simulink model "test_dynamics_sim"  (R2021b)
settings: Solver=ode8  StartTime=0.0  StopTime=5000  FixedStep=0.01  RelTol=1e-3
values from neighbouring files (symbols this model uses):
  invJ = inv(J)    [test_dynamics1.m]    (also in test_dynamics2.m)
  Ir = 0    [test_dynamics1.m]    (also in test_dynamics2.m = 0.005)
  Ix = 0.0504    [test_dynamics1.m]    (also in test_dynamics2.m = 0.01)
  Iy = 0.0504    [test_dynamics1.m]    (also in test_dynamics2.m = 0.05)
  Iz = 0.0109    [test_dynamics1.m]    (also in test_dynamics2.m = 0.07)
  J = [Ix 0 0; 0 Iy 0; 0 0 Iz]    [test_dynamics1.m]    (also in test_dynamics2.m)
  Mx = 0    [test_dynamics2.m]
  My = 0    [test_dynamics2.m]
  Mz = 0    [test_dynamics2.m]
  omega0 = [omegax0, omegay0, omegaz0]'    [test_dynamics1.m]    (also in test_dynamics2.m)
  omegar = 0    [test_dynamics1.m]    (also in test_dynamics2.m = 6.28318530718)
  omegax0 = 0.45    [test_dynamics1.m]    (also in test_dynamics2.m = 1e-06)
  omegay0 = 0.52    [test_dynamics1.m]    (also in test_dynamics2.m = 1e-06)
  omegaz0 = 0.55    [test_dynamics1.m]    (also in test_dynamics2.m = 0.02)
  T_w = [0 0 0.0004]'    [test_dynamics2.m]
libraries: my_math_ops x3, vrlib x1
settings Model: Creator=Davide  LastModifiedBy=Davide
settings SolverCC: AlgebraicLoopSolver=TrustRegion
settings DebuggingCC: SFMachineParentedDataDiag=warning

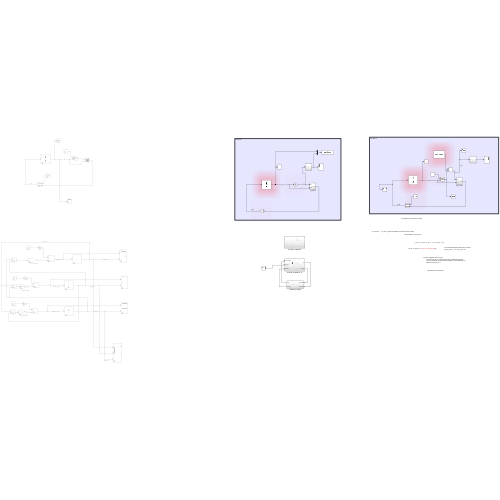
[thumbnail: Simulink's stored preview of the top-level diagram]
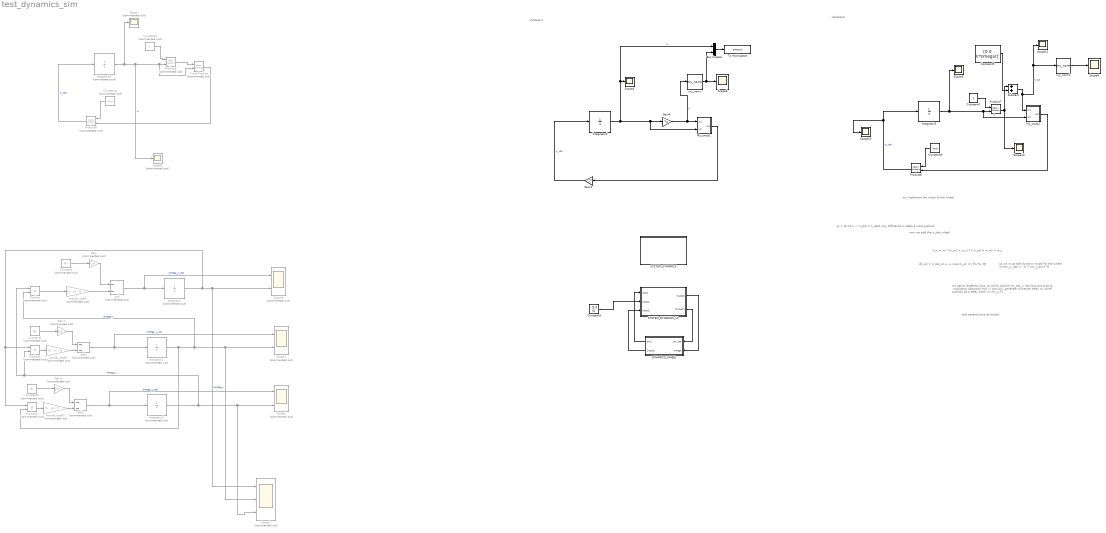
== system test_dynamics_sim ==
  note: Validator2
  note: Validator1
  note: add square wave as torque
  note: we get an algebraic loop, to solve:
      | explicit om_dot_z, rewriting but loosing ,modularity approach
      | trick in simulink, generate numerical delay on some quantity as a
      | delay block on om_z Z-1
  note: so we must add dynamic model for the wheel
      | Iw*om_w_dot = - Iw * om_z_dot + M
  note: dh_wh = h_dot_wh + w cross h_wh = [ Rx Ry M]
  note: h_w = Iw * (w_wh + w_z) * k w_rel = w_wh + w_z
  note: now we add the w_dot_wheel
  note: try implement the wdotr of the wheel
  note: Jw + I0 w0 k -> h_dot = h_dot0 only difference in relative cross product
  Add : Sum  Commented=on  Inputs=--
  Add1 : Sum  Commented=on  Inputs=--
  Add2 : Sum  Commented=on  Inputs=--
  Bus Creator : BusCreator  Inputs=2
  Constant : Constant  Commented=on  Value=Mx
  Constant1 : Constant  Commented=on  Value=My
  Constant2 : Constant  Commented=on  Value=Mz
  Constant3 : Constant  Commented=on  Value=J
  Constant4 : Constant  Commented=on  Value=invJ
  Constant5 : Constant  Value=[0 0 0]'
  Constant7 : Constant  Value=J
  Constant8 : Constant  Value=invJ
  Constant9 : Constant  Value=[0 0 Ir*omegar]'
  Cross Product : vrlib/Utilities/Cross Product  Commented=on
  DYNAMICS_WHEEL : Subsystem
  Gain : Gain  Commented=on  Gain=1/Ix
  Gain1 : Gain  Commented=on  Gain=1/Iy
  Gain2 : Gain  Commented=on  Gain=1/Iz
  Gain3 : Gain  Gain=invJ  Multiplication=Matrix(K*u)
  Gain4 : Gain  Gain=J  Multiplication=Matrix(K*u)
  Inertial_coeff : Gain  Commented=on  Gain=(Iy - Iz) / Ix
  Inertial_coeff1 : Gain  Commented=on  Gain=(Iz - Ix) / Iy
  Inertial_coeff2 : Gain  Commented=on  Gain=(Ix - Iy) / Iz
  Integrator : Integrator  Commented=on  InitialCondition=omegax0
  Integrator1 : Integrator  Commented=on  InitialCondition=omegay0
  Integrator2 : Integrator  Commented=on  InitialCondition=omegaz0
  Integrator3 : Integrator  Commented=on  InitialCondition=omega0
  Integrator4 : Integrator  InitialCondition=omega0
  Integrator5 : Integrator  InitialCondition=omega0
  My_cross1 : Subsystem
  My_cross2 : Subsystem
  Product : Product  Commented=on
  Product1 : Product  Commented=on
  Product2 : Product  Commented=on
  Product3 : Product  Commented=on  Multiplication=Matrix(*)
  Product4 : Product  Commented=on  Multiplication=Matrix(*)
  Product7 : Product  Multiplication=Matrix(*)
  Product8 : Product  Multiplication=Matrix(*)
  SYSTEM_DYNAMICS : Subsystem
  SYSTEM_DYNAMICS_V2 : Subsystem
  Scope : Scope  Commented=on
  Scope1 : Scope  Commented=on  NumInputPorts=2
  Scope{4..5,8..12} (7 alike) : Scope
  Scope2 : Scope  Commented=on  NumInputPorts=2
  Scope3 : Scope  Commented=on  NumInputPorts=2
  Scope6 : Scope  Commented=on
  Scope7 : Scope  Commented=on  NumInputPorts=3
  Subtract : Sum
  To Workspace : ToWorkspace  VariableName=simout  SampleTime=-1
  my_norm : my_math_ops/my_norm  SystemSampleTime=-1  VariantActivationTime=update diagram  Latency=0  AutoFrameSizeCalculation=off
  my_norm1 : my_math_ops/my_norm  SystemSampleTime=-1  VariantActivationTime=update diagram  Latency=0  AutoFrameSizeCalculation=off
  wires:
  Add/1 -> Scope3/1, Integrator/1  "omega_x_dot"
  Integrator/1 -> Scope7/1, Scope3/2, Product2/1, Product1/1  "omega_x"
  Integrator1/1 -> Product2/2, Scope7/2, Scope1/2, Product/2  "omega_y"
  Add1/1 -> Scope1/1, Integrator1/1  "omega_y_dot"
  Integrator2/1 -> Scope7/3, Scope2/2, Product1/2, Product/1  "omega_z"
  Add2/1 -> Scope2/1, Integrator2/1  "omega_z_dot"
  Product/1 -> Inertial_coeff/1
  Inertial_coeff/1 -> Add/2
  Constant/1 -> Gain/1
  Gain/1 -> Add/1
  Constant1/1 -> Gain1/1
  Gain1/1 -> Add1/1
  Product1/1 -> Inertial_coeff1/1
  Inertial_coeff1/1 -> Add1/2
  Gain2/1 -> Add2/1
  Product2/1 -> Inertial_coeff2/1
  Constant2/1 -> Gain2/1
  Inertial_coeff2/1 -> Add2/2
  Integrator3/1 -> Scope/1, Scope6/1, Product3/2, Cross Product/2  "w"
  Product3/1 -> Cross Product/1
  Cross Product/1 -> Product4/2
  Constant3/1 -> Product3/1
  Constant4/1 -> Product4/1
  Product4/1 -> Integrator3/1  "w_dot"
  Gain4/1 -> My_cross1/1(w1), my_norm/1  "h"
  Integrator4/1 -> Bus Creator/1, Scope4/1, My_cross1/2(w2), Gain4/1  "w"
  Gain3/1 -> Integrator4/1  "w_dot"
  My_cross1/1(w3) -> Gain3/1
  My_cross2/1(w3) -> Product8/2
  Constant7/1 -> Product7/1
  Integrator5/1 -> Scope5/1, My_cross2/2(w2), Product7/2  "w"
  Constant8/1 -> Product8/1
  Product8/1 -> Scope10/1, Integrator5/1  "w_dot"
  Constant9/1 -> Subtract/2
  Product7/1 -> Scope12/1, Subtract/1
  Subtract/1 -> my_norm1/1, Scope11/1, My_cross2/1(w1)  "h_tot"
  my_norm/1 -> Bus Creator/2, Scope8/1
  my_norm1/1 -> Scope9/1
  Bus Creator/1 -> To Workspace/1
  SYSTEM_DYNAMICS_V2/2(Output1) -> DYNAMICS_WHEEL/1(om_dot)
  SYSTEM_DYNAMICS_V2/1(Output) -> DYNAMICS_WHEEL/2(omega)
  DYNAMICS_WHEEL/1(om_r) -> SYSTEM_DYNAMICS_V2/1(Input)
  Constant5/1 -> SYSTEM_DYNAMICS_V2/2(Input2)
  DYNAMICS_WHEEL/2(Output) -> SYSTEM_DYNAMICS_V2/3(Input3)

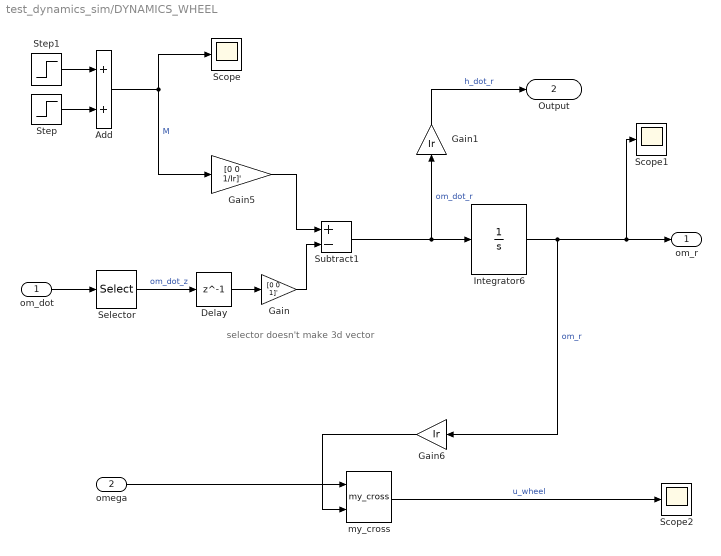
== system test_dynamics_sim/DYNAMICS_WHEEL ==
  note: selector doesn't make 3d vector
  om_dot : Inport
  omega : Inport  Port=2
  Add : Sum
  Delay : Delay  DelayLength=1
  Gain : Gain  Gain=[0 0 1]'
  Gain1 : Gain  Gain=Ir
  Gain5 : Gain  Gain=[0 0 1/Ir]'
  Gain6 : Gain  Gain=Ir
  Integrator6 : Integrator  InitialCondition=[0 0 0]'
  Scope : Scope
  Scope1 : Scope
  Scope2 : Scope
  Selector : Selector  InputPortWidth=3  IndexOptions=Index vector (dialog)  Indices=3  OutputSizes=1
  Step : Step  Time=255  After=-T_w  SampleTime=0
  Step1 : Step  Time=250  After=T_w  SampleTime=0
  Subtract1 : Sum  Inputs=+-
  my_cross : my_math_ops/my_cross  SystemSampleTime=-1  VariantActivationTime=update diagram  Latency=0  AutoFrameSizeCalculation=off
  om_r : Outport
  Output : Outport  Port=2
  wires:
  Selector/1 -> Delay/1  "om_dot_z"
  Add/1 -> Scope/1, Gain5/1  "M"
  omega/1 -> my_cross/1
  om_dot/1 -> Selector/1
  Gain6/1 -> my_cross/2
  Integrator6/1 -> Scope1/1, om_r/1, Gain6/1  "om_r"
  Gain5/1 -> Subtract1/1
  Subtract1/1 -> Gain1/1, Integrator6/1  "om_dot_r"
  my_cross/1 -> Scope2/1  "u_wheel"
  Step1/1 -> Add/1
  Step/1 -> Add/2
  Delay/1 -> Gain/1
  Gain/1 -> Subtract1/2
  Gain1/1 -> Output/1  "h_dot_r"

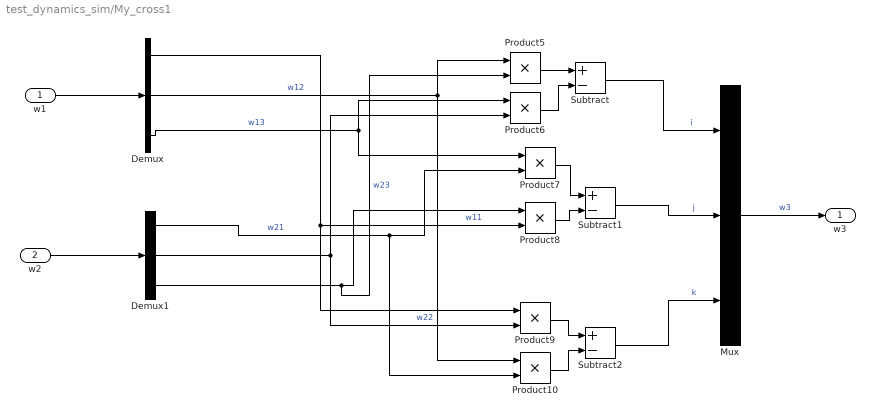
== system test_dynamics_sim/My_cross1 ==
  w1 : Inport
  w2 : Inport  Port=2
  Demux : Demux  Outputs=3
  Demux1 : Demux  Outputs=3
  Mux : Mux  Inputs=3
  Product{5..10} (6 alike) : Product
  Subtract : Sum  Inputs=+-
  Subtract1 : Sum  Inputs=+-
  Subtract2 : Sum  Inputs=+-
  w3 : Outport
  wires:
  Subtract1/1 -> Mux/2  "j"
  Product6/1 -> Subtract/2
  Demux1/3 -> Product5/2, Product8/1  "w23"
  Demux/1 -> Product9/1, Product8/2  "w11"
  Demux/3 -> Product7/1, Product6/1  "w13"
  Product5/1 -> Subtract/1
  Demux1/1 -> Product10/2, Product7/2  "w21"
  Product9/1 -> Subtract2/1
  Demux1/2 -> Product9/2, Product6/2  "w22"
  Demux/2 -> Product5/1, Product10/1  "w12"
  Subtract/1 -> Mux/1  "i"
  w2/1 -> Demux1/1
  Product10/1 -> Subtract2/2
  Product7/1 -> Subtract1/1
  Product8/1 -> Subtract1/2
  Subtract2/1 -> Mux/3  "k"
  w1/1 -> Demux/1
  Mux/1 -> w3/1  "w3"

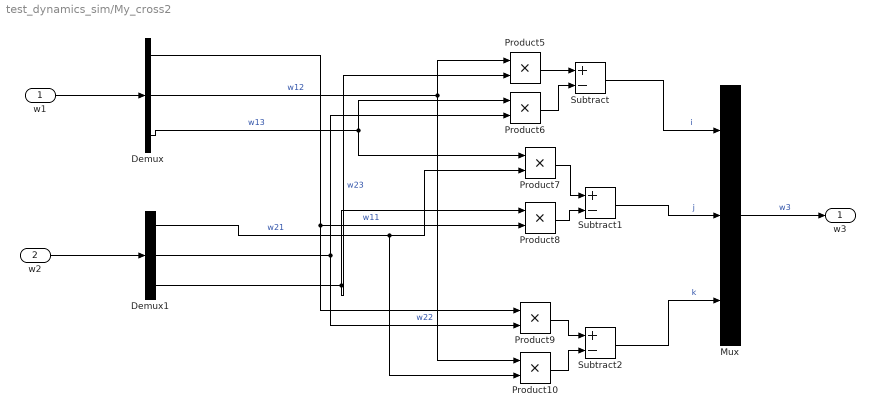
== system test_dynamics_sim/My_cross2 ==
  w1 : Inport
  w2 : Inport  Port=2
  Demux : Demux  Outputs=3
  Demux1 : Demux  Outputs=3
  Mux : Mux  Inputs=3
  Product{5..10} (6 alike) : Product
  Subtract : Sum  Inputs=+-
  Subtract1 : Sum  Inputs=+-
  Subtract2 : Sum  Inputs=+-
  w3 : Outport
  wires:
  Subtract1/1 -> Mux/2  "j"
  Product6/1 -> Subtract/2
  Demux1/3 -> Product5/2, Product8/1  "w23"
  Demux/1 -> Product9/1, Product8/2  "w11"
  Demux/3 -> Product7/1, Product6/1  "w13"
  Product5/1 -> Subtract/1
  Demux1/1 -> Product10/2, Product7/2  "w21"
  Product9/1 -> Subtract2/1
  Demux1/2 -> Product9/2, Product6/2  "w22"
  Demux/2 -> Product5/1, Product10/1  "w12"
  Subtract/1 -> Mux/1  "i"
  w2/1 -> Demux1/1
  Product10/1 -> Subtract2/2
  Product7/1 -> Subtract1/1
  Product8/1 -> Subtract1/2
  Subtract2/1 -> Mux/3  "k"
  w1/1 -> Demux/1
  Mux/1 -> w3/1  "w3"

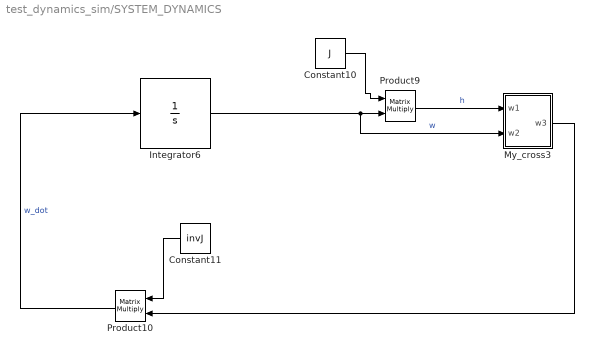
== system test_dynamics_sim/SYSTEM_DYNAMICS ==
  Constant10 : Constant  Value=J
  Constant11 : Constant  Value=invJ
  Integrator6 : Integrator  InitialCondition=omega0
  My_cross3 : Subsystem
  Product10 : Product  Multiplication=Matrix(*)
  Product9 : Product  Multiplication=Matrix(*)
  wires:
  Integrator6/1 -> My_cross3/2(w2), Product9/2  "w"
  Constant10/1 -> Product9/1
  Constant11/1 -> Product10/1
  Product9/1 -> My_cross3/1(w1)  "h"
  My_cross3/1(w3) -> Product10/2
  Product10/1 -> Integrator6/1  "w_dot"

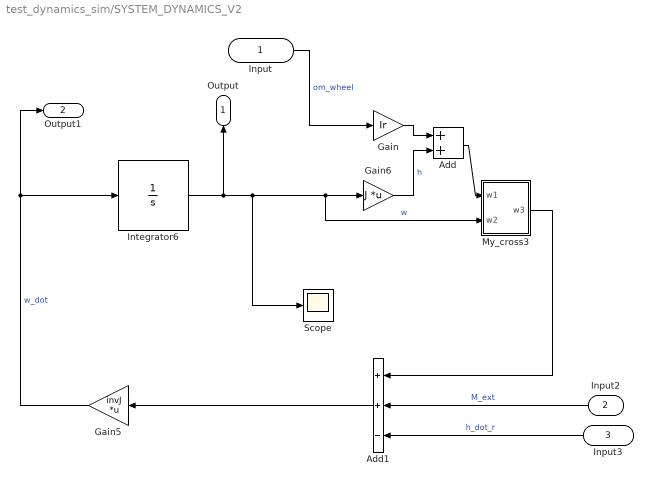
== system test_dynamics_sim/SYSTEM_DYNAMICS_V2 ==
  Input : Inport
  Input2 : Inport  Port=2
  Input3 : Inport  Port=3
  Add : Sum
  Add1 : Sum  Inputs=++-
  Gain : Gain  Gain=Ir
  Gain5 : Gain  Gain=invJ  Multiplication=Matrix(K*u)
  Gain6 : Gain  Gain=J  Multiplication=Matrix(K*u)
  Integrator6 : Integrator  InitialCondition=omega0
  My_cross3 : Subsystem
  Scope : Scope
  Output : Outport
  Output1 : Outport  Port=2
  wires:
  Gain6/1 -> Add/2  "h"
  Integrator6/1 -> Output/1, Scope/1, My_cross3/2(w2), Gain6/1  "w"
  Gain5/1 -> Output1/1, Integrator6/1  "w_dot"
  Gain/1 -> Add/1
  Add/1 -> My_cross3/1(w1)
  Input/1 -> Gain/1  "om_wheel"
  Add1/1 -> Gain5/1
  My_cross3/1(w3) -> Add1/1
  Input3/1 -> Add1/3  "h_dot_r"
  Input2/1 -> Add1/2  "M_ext"

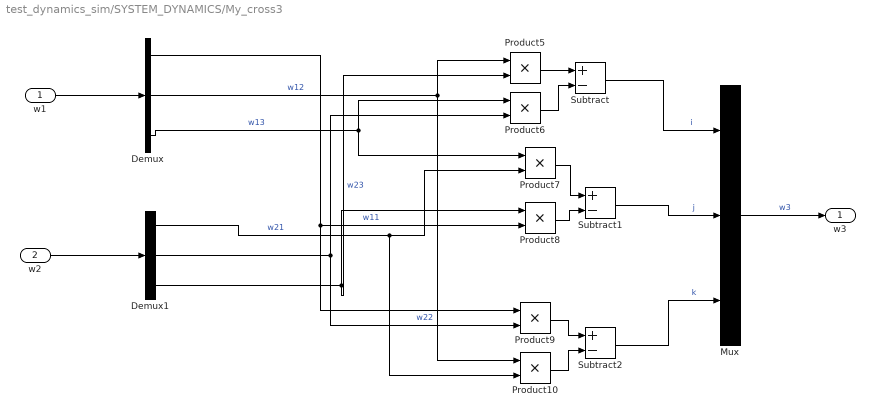
== system test_dynamics_sim/SYSTEM_DYNAMICS/My_cross3 ==
  w1 : Inport
  w2 : Inport  Port=2
  Demux : Demux  Outputs=3
  Demux1 : Demux  Outputs=3
  Mux : Mux  Inputs=3
  Product{5..10} (6 alike) : Product
  Subtract : Sum  Inputs=+-
  Subtract1 : Sum  Inputs=+-
  Subtract2 : Sum  Inputs=+-
  w3 : Outport
  wires:
  Subtract1/1 -> Mux/2  "j"
  Product6/1 -> Subtract/2
  Demux1/3 -> Product5/2, Product8/1  "w23"
  Demux/1 -> Product9/1, Product8/2  "w11"
  Demux/3 -> Product7/1, Product6/1  "w13"
  Product5/1 -> Subtract/1
  Demux1/1 -> Product10/2, Product7/2  "w21"
  Product9/1 -> Subtract2/1
  Demux1/2 -> Product9/2, Product6/2  "w22"
  Demux/2 -> Product5/1, Product10/1  "w12"
  Subtract/1 -> Mux/1  "i"
  w2/1 -> Demux1/1
  Product10/1 -> Subtract2/2
  Product7/1 -> Subtract1/1
  Product8/1 -> Subtract1/2
  Subtract2/1 -> Mux/3  "k"
  w1/1 -> Demux/1
  Mux/1 -> w3/1  "w3"

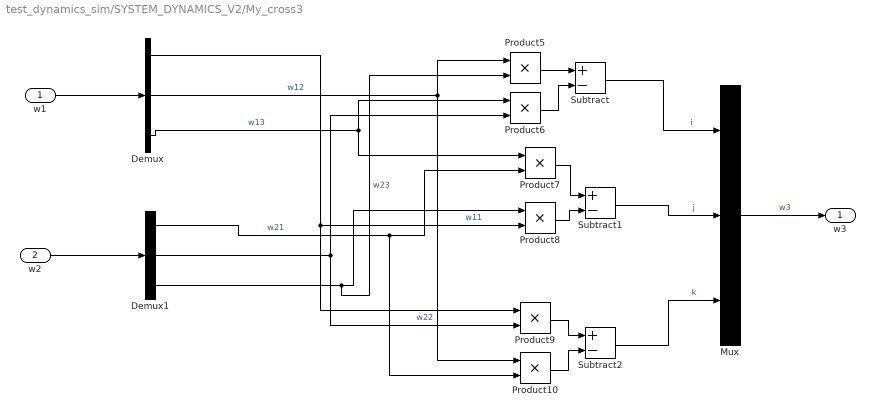
== system test_dynamics_sim/SYSTEM_DYNAMICS_V2/My_cross3 ==
  w1 : Inport
  w2 : Inport  Port=2
  Demux : Demux  Outputs=3
  Demux1 : Demux  Outputs=3
  Mux : Mux  Inputs=3
  Product{5..10} (6 alike) : Product
  Subtract : Sum  Inputs=+-
  Subtract1 : Sum  Inputs=+-
  Subtract2 : Sum  Inputs=+-
  w3 : Outport
  wires:
  Subtract1/1 -> Mux/2  "j"
  Product6/1 -> Subtract/2
  Demux1/3 -> Product5/2, Product8/1  "w23"
  Demux/1 -> Product9/1, Product8/2  "w11"
  Demux/3 -> Product7/1, Product6/1  "w13"
  Product5/1 -> Subtract/1
  Demux1/1 -> Product10/2, Product7/2  "w21"
  Product9/1 -> Subtract2/1
  Demux1/2 -> Product9/2, Product6/2  "w22"
  Demux/2 -> Product5/1, Product10/1  "w12"
  Subtract/1 -> Mux/1  "i"
  w2/1 -> Demux1/1
  Product10/1 -> Subtract2/2
  Product7/1 -> Subtract1/1
  Product8/1 -> Subtract1/2
  Subtract2/1 -> Mux/3  "k"
  w1/1 -> Demux/1
  Mux/1 -> w3/1  "w3"
